simulink model "sampleModel1627"  (R2023a)
settings: Solver=VariableStepAuto  StartTime=0.0  StopTime=10.0  RelTol=1e-3
libraries: hdlsllib x3, simulink x2
settings Model: Creator=user1  LastModifiedBy=user1

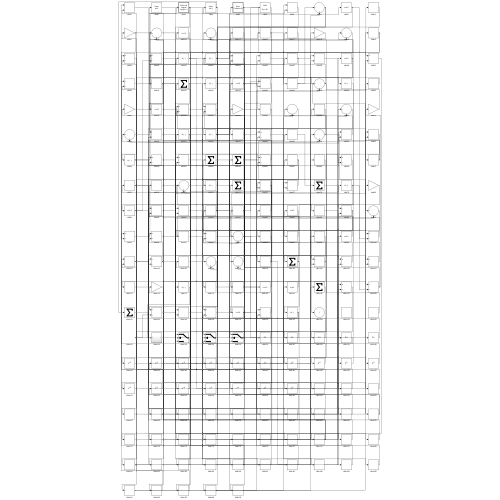
[thumbnail: Simulink's stored preview of the top-level diagram]
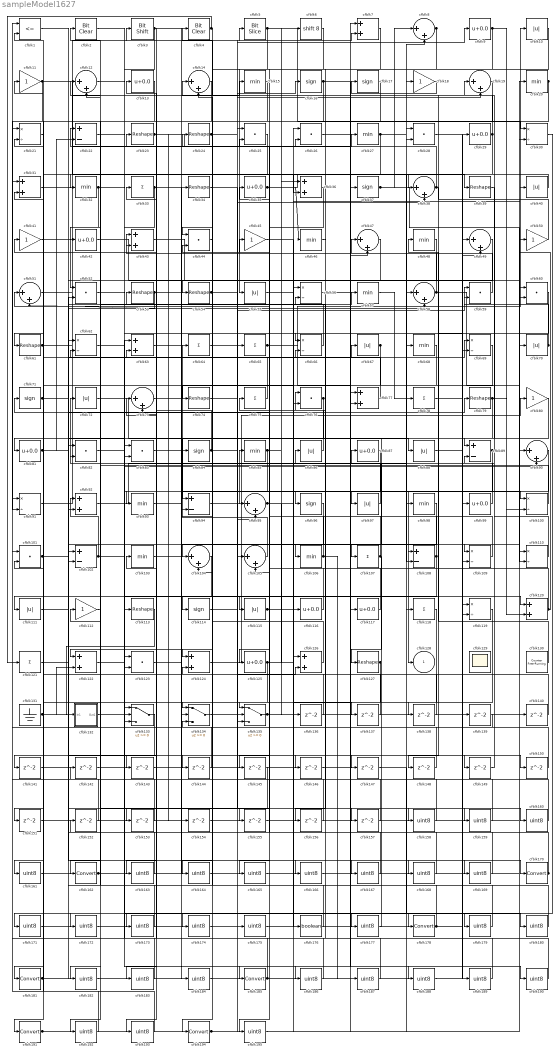
== system sampleModel1627 ==
  cfblk1 : RelationalOperator  Operator=<=  OutDataTypeStr=boolean  InputSameDT=off
  cfblk{10,40,55,67,70,72,86,88,97,111,115} (11 alike) : Abs  SaturateOnIntegerOverflow=off
  cfblk{21,30,56,62,66,69,91,100,109..110,119} (11 alike) : Product  Inputs=*/  RndMeth=Zero  SaturateOnIntegerOverflow=on
  cfblk{25..26,28,44,52,59..60,76,82..83,101,123} (12 alike) : DotProduct  OutDataTypeStr=Inherit: Inherit via internal rule
  cfblk{22,89,94,102,108} (5 alike) : Sum  Inputs=+-
  cfblk{15,20,27,32,46,48,57,68,85,93,98,103,106} (13 alike) : MinMax
  cfblk{8,12,14,19,38,47,49,51,58,73,90,95,104..105} (14 alike) : Sum  Inputs=|++
  cfblk{33,64..65,75,78,107,118,121} (8 alike) : Sum  Inputs=+
  cfblk{11,18,41,45,50,80,112} (7 alike) : Gain
  cfblk{23..24,34,39,53..54,61,74,79,113,127} (11 alike) : Reshape
  cfblk{16..17,37,71,84,96,114} (7 alike) : Signum
  cfblk{9,13,29,35,42,81,87,99,116..117,125} (11 alike) : Bias  Bias=0.0  SaturateOnIntegerOverflow=off
  cfblk{7,31,36,43,63,77,92,120,122,124,126} (11 alike) : Sum
  cfblk129 : Scope
      settings: Floating=on
  cfblk130 : hdlsllib/Sources/Counter Free-Running  NumBits=16  tsamp=-1
  cfblk131 : Ground
  cfblk132 : Subsystem
      settings: LibrarySourceBlock=|
      | hdlsllib/Ports &
      | Subsystems/Subsystem
  cfblk133 : Switch  SaturateOnIntegerOverflow=off  InputSameDT=off
  cfblk134 : Switch  SaturateOnIntegerOverflow=off  InputSameDT=off
  cfblk135 : Switch  SaturateOnIntegerOverflow=off  InputSameDT=off
  cfblk{136..157} (22 alike) : Delay  SampleTime=1
  cfblk{158..161,163..169,171..175,177,179..180,182..184,186..190,192..193,195} (30 alike) : DataTypeConversion  OutDataTypeStr=uint8  SaturateOnIntegerOverflow=off  RndMeth=Floor
  cfblk{162,170,178,181,185,191,194} (7 alike) : DataTypeConversion  SaturateOnIntegerOverflow=off  RndMeth=Floor
  cfblk176 : DataTypeConversion  OutDataTypeStr=boolean  SaturateOnIntegerOverflow=off  RndMeth=Floor
  cfblk2 : simulink/Logic and Bit Operations/Bit Clear  iBit=0
      settings: LibrarySourceBlock=|
      | hdlsllib/Logic and Bit
      | Operations/Bit Clear
  cfblk3 : hdlsllib/Logic and Bit Operations/Bit Shift  mode=Shift Left Logical  N=0
  cfblk4 : simulink/Logic and Bit Operations/Bit Clear  iBit=0
      settings: LibrarySourceBlock=|
      | hdlsllib/Logic and Bit
      | Operations/Bit Clear
  cfblk5 : hdlsllib/Logic and Bit Operations/Bit Slice  lidx=7  ridx=0
  cfblk6 : ArithShift  BitShiftNumber=8
  cfblk128 : Outport  VectorParamsAs1DForOutWhenUnconnected=off
  wires:
  cfblk19/1 -> cfblk122/1
  cfblk59/1 -> cfblk43/1
  cfblk124/1 -> cfblk80/1
  cfblk73/1 -> cfblk185/1
  cfblk98/1 -> cfblk194/1
  cfblk57/1 -> cfblk78/1
  cfblk21/1 -> cfblk191/1
  cfblk70/1 -> cfblk10/1, cfblk19/1
  cfblk113/1 -> cfblk132/1(In1)
  cfblk84/1 -> cfblk41/1, cfblk9/1, cfblk59/2
  cfblk23/1 -> cfblk26/2, cfblk154/1
  cfblk75/1 -> cfblk33/1
  cfblk94/1 -> cfblk85/1
  cfblk31/1 -> cfblk27/1
  cfblk130/1 -> cfblk48/1
  cfblk37/1 -> cfblk90/1, cfblk8/1
  cfblk105/1 -> cfblk64/1
  cfblk32/1 -> cfblk109/1, cfblk52/1, cfblk66/1
  cfblk64/1 -> cfblk95/1
  cfblk81/1 -> cfblk22/2, cfblk157/1
  cfblk67/1 -> cfblk92/2, cfblk156/1
  cfblk51/1 -> cfblk3/1
  cfblk50/1 -> cfblk14/1
  cfblk61/1 -> cfblk5/1, cfblk63/2
  cfblk112/1 -> cfblk162/1
  cfblk63/1 -> cfblk97/1
  cfblk9/1 -> cfblk55/1, cfblk120/2
  cfblk96/1 -> cfblk104/1
  cfblk44/1 -> cfblk114/1
  cfblk48/1 -> cfblk102/2
  cfblk127/1 -> cfblk135/1, cfblk124/2
  cfblk47/1 -> cfblk134/1
  cfblk90/1 -> cfblk128/1
  cfblk13/1 -> cfblk81/1
  cfblk115/1 -> cfblk69/1, cfblk150/1
  cfblk8/1 -> cfblk54/1, cfblk195/1
  cfblk117/1 -> cfblk53/1
  cfblk27/1 -> cfblk61/1, cfblk8/2
  cfblk65/1 -> cfblk60/1, cfblk77/2
  cfblk46/1 -> cfblk106/1
  cfblk41/1 -> cfblk23/1
  cfblk131/1 -> cfblk79/1, cfblk122/2
  cfblk7/1 -> cfblk96/1
  cfblk106/1 -> cfblk45/1, cfblk44/2, cfblk187/1
  cfblk54/1 -> cfblk88/1, cfblk19/2, cfblk38/2
  cfblk91/1 -> cfblk15/1
  cfblk132/1(Out1) -> cfblk67/1
  cfblk97/1 -> cfblk72/1
  cfblk5/1 -> cfblk30/1, cfblk44/1
  cfblk16/1 -> cfblk37/1, cfblk42/1
  cfblk55/1 -> cfblk40/1
  cfblk40/1 -> cfblk32/1
  cfblk79/1 -> cfblk107/1, cfblk100/2
  cfblk108/1 -> cfblk111/1, cfblk66/2
  cfblk110/1 -> cfblk59/1
  cfblk12/1 -> cfblk83/1
  cfblk11/1 -> cfblk39/1, cfblk91/2
  cfblk62/1 -> cfblk178/1
  cfblk85/1 -> cfblk135/2, cfblk6/1
  cfblk86/1 -> cfblk35/1
  cfblk42/1 -> cfblk70/1
  cfblk28/1 -> cfblk170/1
  cfblk66/1 -> cfblk12/1
  cfblk102/1 -> cfblk92/1, cfblk90/2
  cfblk3/1 -> cfblk76/2, cfblk123/2, cfblk193/1
  cfblk122/1 -> cfblk113/1
  cfblk76/1 -> cfblk94/1, cfblk155/1
  cfblk101/1 -> cfblk110/2, cfblk166/1
  cfblk120/1 -> cfblk50/1, cfblk22/1
  cfblk107/1 -> cfblk127/1, cfblk25/2
  cfblk109/1 -> cfblk51/1
  cfblk77/1 -> cfblk31/2
  cfblk10/1 -> cfblk104/2
  cfblk100/1 -> cfblk12/2
  cfblk135/1 -> cfblk20/1, cfblk169/1
  cfblk89/1 -> cfblk93/1, cfblk163/1
  cfblk20/1 -> cfblk125/1, cfblk115/1
  cfblk72/1 -> cfblk95/2
  cfblk39/1 -> cfblk89/1
  cfblk35/1 -> cfblk46/1, cfblk38/1
  cfblk53/1 -> cfblk51/2, cfblk69/2
  cfblk52/1 -> cfblk120/1
  cfblk134/1 -> cfblk126/2
  cfblk4/1 -> cfblk121/1, cfblk74/1
  cfblk24/1 -> cfblk7/2, cfblk16/1
  cfblk118/1 -> cfblk181/1
  cfblk99/1 -> cfblk76/1
  cfblk74/1 -> cfblk100/1
  cfblk18/1 -> cfblk17/1
  cfblk116/1 -> cfblk71/1
  cfblk33/1 -> cfblk108/1, cfblk133/3
  cfblk125/1 -> cfblk36/1, cfblk149/1, cfblk174/1
  cfblk126/1 -> cfblk24/1
  cfblk87/1 -> cfblk133/2
  cfblk95/1 -> cfblk136/1, cfblk137/1
  cfblk111/1 -> cfblk57/1
  cfblk38/1 -> cfblk14/2, cfblk148/1
  cfblk58/1 -> cfblk110/1, cfblk47/1
  cfblk43/1 -> cfblk105/1
  cfblk1/1 -> cfblk58/2
  cfblk92/1 -> cfblk18/1
  cfblk29/1 -> cfblk4/1, cfblk108/2, cfblk36/2
  cfblk25/1 -> cfblk124/1
  cfblk71/1 -> cfblk83/2, cfblk168/1
  cfblk136/1 -> cfblk43/2
  cfblk137/1 -> cfblk105/2
  cfblk60/1 -> cfblk138/1
  cfblk138/1 -> cfblk126/1
  cfblk78/1 -> cfblk139/1
  cfblk139/1 -> cfblk134/3
  cfblk140/1 -> cfblk101/2
  cfblk133/1 -> cfblk141/1
  cfblk141/1 -> cfblk58/1
  cfblk142/1 -> cfblk47/2
  cfblk17/1 -> cfblk143/1
  cfblk121/1 -> cfblk144/1
  cfblk144/1 -> cfblk1/1
  cfblk36/1 -> cfblk145/1
  cfblk114/1 -> cfblk146/1
  cfblk146/1 -> cfblk7/1
  cfblk123/1 -> cfblk147/1
  cfblk148/1 -> cfblk77/1
  cfblk149/1 -> cfblk89/2
  cfblk150/1 -> cfblk134/2
  cfblk69/1 -> cfblk151/1
  cfblk151/1 -> cfblk135/3
  cfblk152/1 -> cfblk1/2
  cfblk15/1 -> cfblk153/1
  cfblk153/1 -> cfblk91/1
  cfblk154/1 -> cfblk30/2
  cfblk155/1 -> cfblk109/2
  cfblk156/1 -> cfblk31/1
  cfblk157/1 -> cfblk13/1
  cfblk103/1 -> cfblk158/1
  cfblk158/1 -> cfblk123/1
  cfblk26/1 -> cfblk159/1
  cfblk159/1 -> cfblk103/1
  cfblk34/1 -> cfblk160/1
  cfblk160/1 -> cfblk11/1
  cfblk80/1 -> cfblk161/1
  cfblk161/1 -> cfblk34/1
  cfblk162/1 -> cfblk142/1, cfblk116/1
  cfblk163/1 -> cfblk112/1
  cfblk49/1 -> cfblk164/1
  cfblk164/1 -> cfblk140/1
  cfblk6/1 -> cfblk165/1
  cfblk165/1 -> cfblk49/1
  cfblk166/1 -> cfblk49/2
  cfblk82/1 -> cfblk167/1
  cfblk167/1 -> cfblk75/1
  cfblk168/1 -> cfblk82/1
  cfblk169/1 -> cfblk82/2
  cfblk170/1 -> cfblk84/1, cfblk25/1
  cfblk30/1 -> cfblk171/1
  cfblk171/1 -> cfblk28/1
  cfblk145/1 -> cfblk172/1
  cfblk172/1 -> cfblk28/2
  cfblk119/1 -> cfblk173/1
  cfblk173/1 -> cfblk133/1
  cfblk174/1 -> cfblk119/1
  cfblk175/1 -> cfblk119/2
  cfblk45/1 -> cfblk176/1
  cfblk176/1 -> cfblk2/1
  cfblk2/1 -> cfblk177/1
  cfblk177/1 -> cfblk87/1
  cfblk178/1 -> cfblk152/1, cfblk94/2, cfblk86/1
  cfblk147/1 -> cfblk179/1
  cfblk179/1 -> cfblk62/1
  cfblk93/1 -> cfblk180/1
  cfblk180/1 -> cfblk62/2
  cfblk181/1 -> cfblk52/2, cfblk65/1
  cfblk104/1 -> cfblk182/1
  cfblk182/1 -> cfblk118/1
  cfblk68/1 -> cfblk183/1
  cfblk183/1 -> cfblk101/1
  cfblk83/1 -> cfblk184/1
  cfblk184/1 -> cfblk68/1
  cfblk185/1 -> cfblk29/1, cfblk63/1, cfblk102/1
  cfblk143/1 -> cfblk186/1
  cfblk186/1 -> cfblk73/1
  cfblk187/1 -> cfblk73/2
  cfblk56/1 -> cfblk188/1
  cfblk188/1 -> cfblk99/1
  cfblk88/1 -> cfblk189/1
  cfblk189/1 -> cfblk56/1
  cfblk22/1 -> cfblk190/1
  cfblk190/1 -> cfblk56/2
  cfblk191/1 -> cfblk175/1, cfblk26/1
  cfblk14/1 -> cfblk192/1
  cfblk192/1 -> cfblk21/1
  cfblk193/1 -> cfblk21/2
  cfblk194/1 -> cfblk60/2, cfblk117/1
  cfblk195/1 -> cfblk98/1

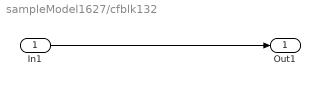
== system sampleModel1627/cfblk132 ==
  In1 : Inport
  Out1 : Outport
  wires:
  In1/1 -> Out1/1
